simulink model "DynamicVibrationAbsorber"  (R2020a)
settings: Solver=VariableStepAuto  StartTime=0.0  StopTime=10  MaxStep=dt  RelTol=1e-3
values from neighbouring files (symbols this model uses):
  b = 50    [ConstantValues.m]
  k1 = 50    [ConstantValues.m]
  M1 = 100    [ConstantValues.m]
settings Model: Creator=DELL  LastModifiedBy=DELL
settings DataIOCC: ExternalInput=[t, sig]  LoadExternalInput=on

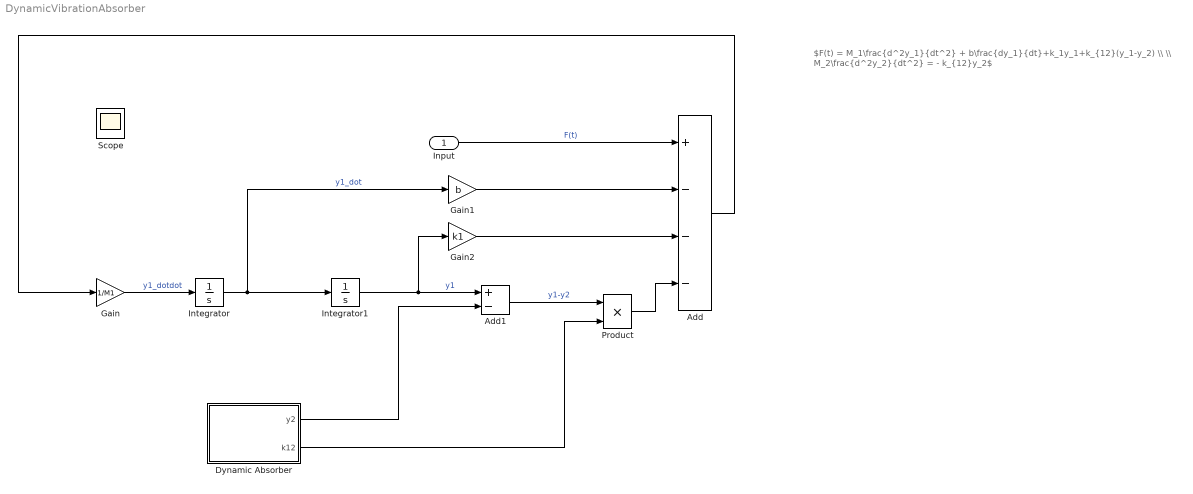
== system DynamicVibrationAbsorber ==
  note: $F(t) = M_1\frac{d^2y_1}{dt^2} + b\frac{dy_1}{dt}+k_1y_1+k_{12}(y_1-y_2) \\ \\ M_2\frac{d^2y_2}{dt^2} = - k_{12}y_2$
  Input : Inport
  Add : Sum  Inputs=+---
  Add1 : Sum  Inputs=+-
  Dynamic Absorber : Subsystem  mask{M2=10, k12=60.0}
      mask prompts: M2 "Mass of Absorber (M2)"; k12 "Stiffness of Absorber (k12)"
      mask DialogControl DescGroupVar Prompt: Dynamic Vibration Absorber Subsystem
      mask DialogControl DescTextVar Prompt: Absorber Parameter
  Gain : Gain  Gain=1/M1
  Gain1 : Gain  Gain=b
  Gain2 : Gain  Gain=k1
  Integrator : Integrator
  Integrator1 : Integrator
  Product : Product
  Scope : Scope
  wires:
  Gain/1 -> Integrator/1  "y1_dotdot"
  Integrator/1 -> Gain1/1, Integrator1/1  "y1_dot"
  Integrator1/1 -> Add1/1, Gain2/1  "y1"
  Add/1 -> Gain/1
  Gain1/1 -> Add/2
  Gain2/1 -> Add/3
  Add1/1 -> Product/1  "y1-y2"
  Product/1 -> Add/4
  Dynamic Absorber/1(y2) -> Add1/2
  Dynamic Absorber/2(k12) -> Product/2
  Input/1 -> Add/1  "F(t)"

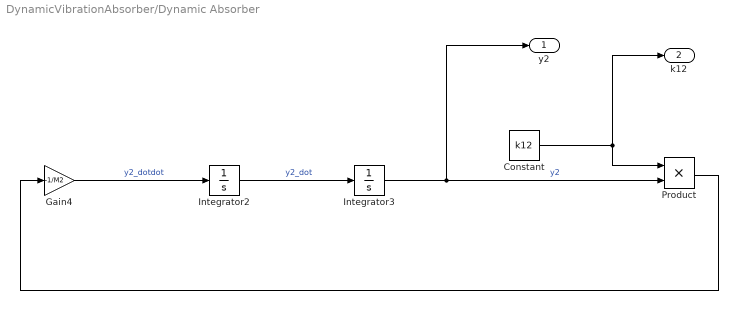
== system DynamicVibrationAbsorber/Dynamic Absorber ==
  Constant : Constant  Value=k12
  Gain4 : Gain  Gain=-1/M2
  Integrator2 : Integrator
  Integrator3 : Integrator
  Product : Product
  y2 : Outport
  k12 : Outport  Port=2
  wires:
  Integrator3/1 -> y2/1, Product/2  "y2"
  Gain4/1 -> Integrator2/1  "y2_dotdot"
  Integrator2/1 -> Integrator3/1  "y2_dot"
  Constant/1 -> k12/1, Product/1
  Product/1 -> Gain4/1
